simulink library "bcm"  (R2021b)
settings: Solver=VariableStepAuto  StartTime=0.0  StopTime=10.0  RelTol=1e-3
undefined symbols (not defined in the file or in its folder): ENUM_ANTITHEFT_ALARM, ENUM_ANTITHEFT_ARM, ENUM_ANTITHEFT_DISARM, ENUM_ANTITHEFT_WAIT, ENUM_GEARPOSNTOCAN_P, ENUM_PDKEYRAWLULOCK_INUNLOCK, ENUM_PDKEYRAWPS_INPS, ENUM_POWERSTA_ON, ENUM_POWERSTA_READY, ENUM_POWERSTA_STANDBY, ENUM_PWRSTASW_ON, ENUM_PWRSTASW_READY, ENUM_VEHICLETYPE_D21, ENUM_VEHICLETYPE_D31F25, ENUM_VEHICLETYPE_D31HAWD, ENUM_VEHICLETYPE_D31HRWD, ENUM_VEHICLETYPE_D31L24, FALSE, KBCM_ACCSwcPrsTmr_s, KBCM_ALMBrightnessDark_enum, KBCM_AmbBlue_enum, KBCM_AmbBreathT_ms, KBCM_AmbGreen_enum, KBCM_AmbMidPple_enum, KBCM_AmbRed_enum, KBCM_AmbTempCtrlEN_flg, KBCM_AmbTempT_s, KBCM_AmbWelModeENWait_s, KBCM_Antitheft_enum_ovrdflg, KBCM_Antitheft_enum_ovrdval, KBCM_APMDoorCtrlSta_flg_ovrdflg, KBCM_APMDoorCtrlSta_flg_ovrdval, KBCM_CmdKeepT_s, KBCM_CSWLightRstDebT_s, KBCM_CSWTurnLPRstT_s, KBCM_DelayTSW_flg, KBCM_DiagDRLOFF_flg, KBCM_DiagFLTC_mA, KBCM_DiagFMHT_s, KBCM_DiagFRTC_mA, KBCM_DiagRLTC_mA, KBCM_DiagRRTC_mA, KBCM_DrAPMRetryTimes_cnt, KBCM_DrOpenWdwOT_s, KBCM_DrOpenWdwReady_s, KBCM_ESSOffT_ms, KBCM_ESSOnT_ms, KBCM_FDCDKCReDetectT_K, KBCM_FDCDKCUSSFilterT_K, KBCM_HandleLampKeepT_s, KBCM_IVIRstHoldT_ms, KBCM_IVIRstTriggerT_ms, KBCM_ONDelayT_ms, KBCM_RAPSAbnFlashOFFT_ms, KBCM_RAPSAbnFlashONT_ms, KBCM_ReDetectT_K, KBCM_RightHandDriveEN_flg, KBCM_RLSLowSpdFilterT_s, KBCM_RmLampKeep_min, KBCM_RmLpKeyInT_s ... (+37)
libraries: simulink x389, $bdroot x11, hcu_lib x2
(part 7 of 13)

== system bcm/BCM/BCM/Window_Control_Sig_Combine/Driver_Window ==
  note: 0:NoReq
      | 1:BCM
      | 2.IVI
      | 3:DKC
      | 4:CONN
  note: 0:NoReq
      | 1:BCM
      | 2.IVI
      | 3:DKC
      | 4:CONN
  DKCWINCMD : Inport
  IVIWINCMD : Inport  Port=2
  CONNWINCMD : Inport  Port=3
  BCMWINCMD : Inport  Port=4
  Add{,1..3} (4 alike) : Sum  Inputs=-+
  Compare To Constant{,1..3} (4 alike) : simulink/Logic and Bit Operations/Compare To Constant  relop=>  const=0  OutDataTypeStr=boolean
  Constant{,1..3} (4 alike) : Constant  Value=100
  Constant10 : Constant  Value=127
  Constant{11,13,15,17} (4 alike) : Constant  Value=10
  Constant{8,12,14,16,18} (5 alike) : Constant
  Constant4 : Constant  Value=0
  Constant5 : Constant  Value=4
  Constant6 : Constant  Value=2
  Constant7 : Constant  Value=3
  Constant9 : Constant  Value=127
  Data Type Conversion{,1..6} (7 alike) : DataTypeConversion  OutDataTypeStr=uint8
  Data Type Conversion{7..14} (8 alike) : DataTypeConversion  OutDataTypeStr=int8
  Detect Decrease{1..4} (4 alike) : simulink/Logic and Bit Operations/Detect Decrease  vinit=0.0  OutDataTypeStr=boolean
  Multiport Switch : MultiPortSwitch  DataPortOrder=Zero-based contiguous  Inputs=6  DiagnosticForDefault=None  zeroidx=on
  Relational Operator{,1..3} (4 alike) : RelationalOperator  Operator=>  OutDataTypeStr=boolean  RndMeth=Simplest
  Saturation{,1..3} (4 alike) : Saturate  UpperLimit=10  LowerLimit=0
  Switch{,1..7} (8 alike) : Switch  Criteria=u2 > Threshold
  Unit Delay{,1..3} (4 alike) : UnitDelay  SampleTime=-1  HasFrameUpgradeWarning=on
  WINCMD : Outport
  WINReqAP : Outport  Port=2
  wires:
  Constant7/1 -> Data Type Conversion3/1
  CONNWINCMD/1 -> [CONNWINCMD]
  [CONNWINCMD] -> Relational Operator2/1
  Constant5/1 -> Data Type Conversion1/1
  [WINReqAP] -> Multiport Switch/1
  [BCMReq] -> Switch3/2
  Constant10/1 -> Data Type Conversion6/1
  [DKCReq] -> Switch1/2
  Constant9/1 -> Data Type Conversion5/1
  [CONNReq] -> Switch/2
  [DKCWINCMD] -> Multiport Switch/5
  Constant8/1 -> Data Type Conversion4/1
  Data Type Conversion/1 -> Switch/3
  [BCMWINCMD] -> Multiport Switch/3
  Multiport Switch/1 -> WINCMD/1
  Data Type Conversion3/1 -> Switch1/1
  Data Type Conversion1/1 -> Switch/1
  Constant2/1 -> Relational Operator2/2
  Constant4/1 -> Data Type Conversion/1
  Constant3/1 -> Relational Operator3/2
  Data Type Conversion5/1 -> Multiport Switch/2
  DKCWINCMD/1 -> [DKCWINCMD]
  BCMWINCMD/1 -> [BCMWINCMD]
  IVIWINCMD/1 -> [IVIWINCMD]
  Constant/1 -> Relational Operator/2
  [DKCWINCMD] -> Relational Operator/1
  [IVIWINCMD] -> Multiport Switch/4
  [CONNWINCMD] -> Multiport Switch/6
  Constant1/1 -> Relational Operator1/2
  [BCMWINCMD] -> Relational Operator3/1
  Data Type Conversion4/1 -> Switch3/1
  Switch1/1 -> Switch2/3
  Switch/1 -> Switch1/3
  [IVIWINCMD] -> Relational Operator1/1
  Switch3/1 -> [WINReqAP]
  Switch2/1 -> Switch3/3
  Constant6/1 -> Data Type Conversion2/1
  Data Type Conversion2/1 -> Switch2/1
  [IVIReq] -> Switch2/2
  [WINReqAP] -> WINReqAP/1
  Data Type Conversion6/1 -> Multiport Switch/7
  Relational Operator/1 -> Detect Decrease4/1
  Saturation/1 -> Compare To Constant/1, Unit Delay/1
  Constant11/1 -> Data Type Conversion7/1
  Detect Decrease4/1 -> Switch4/2
  Unit Delay/1 -> Add/2
  Add/1 -> Switch4/3
  Data Type Conversion7/1 -> Switch4/1
  Data Type Conversion8/1 -> Add/1
  Constant12/1 -> Data Type Conversion8/1
  Switch4/1 -> Saturation/1
  Compare To Constant/1 -> [DKCReq]
  Compare To Constant1/1 -> [IVIReq]
  Switch5/1 -> Saturation1/1
  Constant14/1 -> Data Type Conversion10/1
  Data Type Conversion10/1 -> Add1/1
  Data Type Conversion9/1 -> Switch5/1
  Add1/1 -> Switch5/3
  Unit Delay1/1 -> Add1/2
  Detect Decrease1/1 -> Switch5/2
  Constant13/1 -> Data Type Conversion9/1
  Saturation1/1 -> Unit Delay1/1, Compare To Constant1/1
  Relational Operator1/1 -> Detect Decrease1/1
  Saturation2/1 -> Compare To Constant2/1, Unit Delay2/1
  Constant15/1 -> Data Type Conversion12/1
  Detect Decrease2/1 -> Switch6/2
  Unit Delay2/1 -> Add2/2
  Add2/1 -> Switch6/3
  Data Type Conversion12/1 -> Switch6/1
  Data Type Conversion11/1 -> Add2/1
  Constant16/1 -> Data Type Conversion11/1
  Switch6/1 -> Saturation2/1
  Compare To Constant2/1 -> [CONNReq]
  Relational Operator2/1 -> Detect Decrease2/1
  Compare To Constant3/1 -> [BCMReq]
  Switch7/1 -> Saturation3/1
  Constant18/1 -> Data Type Conversion13/1
  Data Type Conversion13/1 -> Add3/1
  Data Type Conversion14/1 -> Switch7/1
  Add3/1 -> Switch7/3
  Unit Delay3/1 -> Add3/2
  Detect Decrease3/1 -> Switch7/2
  Constant17/1 -> Data Type Conversion14/1
  Saturation3/1 -> Unit Delay3/1, Compare To Constant3/1
  Relational Operator3/1 -> Detect Decrease3/1

== system bcm/BCM/BCM/Window_Control_Sig_Combine/Passenger_Window ==
  note: 0:NoReq
      | 1:BCM
      | 2.IVI
      | 3:DKC
      | 4:CONN
  note: 0:NoReq
      | 1:BCM
      | 2.IVI
      | 3:DKC
      | 4:CONN
  DKCWINCMD : Inport
  IVIWINCMD : Inport  Port=2
  CONNWINCMD : Inport  Port=3
  BCMWINCMD : Inport  Port=4
  Add{,1..3} (4 alike) : Sum  Inputs=-+
  Compare To Constant{,1..3} (4 alike) : simulink/Logic and Bit Operations/Compare To Constant  relop=>  const=0  OutDataTypeStr=boolean
  Constant{,1..3} (4 alike) : Constant  Value=100
  Constant10 : Constant  Value=127
  Constant{11,13,15,17} (4 alike) : Constant  Value=10
  Constant{8,12,14,16,18} (5 alike) : Constant
  Constant4 : Constant  Value=0
  Constant5 : Constant  Value=4
  Constant6 : Constant  Value=2
  Constant7 : Constant  Value=3
  Constant9 : Constant  Value=127
  Data Type Conversion{,1..6} (7 alike) : DataTypeConversion  OutDataTypeStr=uint8
  Data Type Conversion{7..14} (8 alike) : DataTypeConversion  OutDataTypeStr=int8
  Detect Decrease{1..4} (4 alike) : simulink/Logic and Bit Operations/Detect Decrease  vinit=0.0  OutDataTypeStr=boolean
  Multiport Switch : MultiPortSwitch  DataPortOrder=Zero-based contiguous  Inputs=6  DiagnosticForDefault=None  zeroidx=on
  Relational Operator{,1..3} (4 alike) : RelationalOperator  Operator=>  OutDataTypeStr=boolean  RndMeth=Simplest
  Saturation{,1..3} (4 alike) : Saturate  UpperLimit=10  LowerLimit=0
  Switch{,1..7} (8 alike) : Switch  Criteria=u2 > Threshold
  Unit Delay{,1..3} (4 alike) : UnitDelay  SampleTime=-1  HasFrameUpgradeWarning=on
  WINCMD : Outport
  WINReqAP : Outport  Port=2
  wires:
  Relational Operator3/1 -> Detect Decrease3/1
  Saturation3/1 -> Compare To Constant3/1, Unit Delay3/1
  Constant17/1 -> Data Type Conversion14/1
  Detect Decrease3/1 -> Switch7/2
  Unit Delay3/1 -> Add3/2
  Add3/1 -> Switch7/3
  Data Type Conversion14/1 -> Switch7/1
  Data Type Conversion13/1 -> Add3/1
  Constant18/1 -> Data Type Conversion13/1
  Switch7/1 -> Saturation3/1
  Compare To Constant3/1 -> [BCMReq]
  Relational Operator2/1 -> Detect Decrease2/1
  Compare To Constant2/1 -> [CONNReq]
  Switch6/1 -> Saturation2/1
  Constant16/1 -> Data Type Conversion11/1
  Data Type Conversion11/1 -> Add2/1
  Data Type Conversion12/1 -> Switch6/1
  Add2/1 -> Switch6/3
  Unit Delay2/1 -> Add2/2
  Detect Decrease2/1 -> Switch6/2
  Constant15/1 -> Data Type Conversion12/1
  Saturation2/1 -> Unit Delay2/1, Compare To Constant2/1
  Relational Operator1/1 -> Detect Decrease1/1
  Saturation1/1 -> Compare To Constant1/1, Unit Delay1/1
  Constant13/1 -> Data Type Conversion9/1
  Detect Decrease1/1 -> Switch5/2
  Unit Delay1/1 -> Add1/2
  Add1/1 -> Switch5/3
  Data Type Conversion9/1 -> Switch5/1
  Data Type Conversion10/1 -> Add1/1
  Constant14/1 -> Data Type Conversion10/1
  Switch5/1 -> Saturation1/1
  Compare To Constant1/1 -> [IVIReq]
  Compare To Constant/1 -> [DKCReq]
  Switch4/1 -> Saturation/1
  Constant12/1 -> Data Type Conversion8/1
  Data Type Conversion8/1 -> Add/1
  Data Type Conversion7/1 -> Switch4/1
  Add/1 -> Switch4/3
  Unit Delay/1 -> Add/2
  Detect Decrease4/1 -> Switch4/2
  Constant11/1 -> Data Type Conversion7/1
  Saturation/1 -> Unit Delay/1, Compare To Constant/1
  Relational Operator/1 -> Detect Decrease4/1
  Data Type Conversion6/1 -> Multiport Switch/7
  [WINReqAP] -> WINReqAP/1
  [IVIReq] -> Switch2/2
  Data Type Conversion2/1 -> Switch2/1
  Constant6/1 -> Data Type Conversion2/1
  Switch2/1 -> Switch3/3
  Switch3/1 -> [WINReqAP]
  [IVIWINCMD] -> Relational Operator1/1
  Switch/1 -> Switch1/3
  Switch1/1 -> Switch2/3
  Data Type Conversion4/1 -> Switch3/1
  [BCMWINCMD] -> Relational Operator3/1
  Constant1/1 -> Relational Operator1/2
  [CONNWINCMD] -> Multiport Switch/6
  [IVIWINCMD] -> Multiport Switch/4
  [DKCWINCMD] -> Relational Operator/1
  Constant/1 -> Relational Operator/2
  IVIWINCMD/1 -> [IVIWINCMD]
  BCMWINCMD/1 -> [BCMWINCMD]
  DKCWINCMD/1 -> [DKCWINCMD]
  Data Type Conversion5/1 -> Multiport Switch/2
  Constant3/1 -> Relational Operator3/2
  Constant4/1 -> Data Type Conversion/1
  Constant2/1 -> Relational Operator2/2
  Data Type Conversion1/1 -> Switch/1
  Data Type Conversion3/1 -> Switch1/1
  Multiport Switch/1 -> WINCMD/1
  [BCMWINCMD] -> Multiport Switch/3
  Data Type Conversion/1 -> Switch/3
  Constant8/1 -> Data Type Conversion4/1
  [DKCWINCMD] -> Multiport Switch/5
  [CONNReq] -> Switch/2
  Constant9/1 -> Data Type Conversion5/1
  [DKCReq] -> Switch1/2
  Constant10/1 -> Data Type Conversion6/1
  [BCMReq] -> Switch3/2
  [WINReqAP] -> Multiport Switch/1
  Constant5/1 -> Data Type Conversion1/1
  [CONNWINCMD] -> Relational Operator2/1
  CONNWINCMD/1 -> [CONNWINCMD]
  Constant7/1 -> Data Type Conversion3/1

== system bcm/BCM/BCM/Window_Control_Sig_Combine/RearLeft_Window ==
  note: 0:NoReq
      | 1:BCM
      | 2.IVI
      | 3:DKC
      | 4:CONN
  note: 0:NoReq
      | 1:BCM
      | 2.IVI
      | 3:DKC
      | 4:CONN
  DKCWINCMD : Inport
  IVIWINCMD : Inport  Port=2
  CONNWINCMD : Inport  Port=3
  BCMWINCMD : Inport  Port=4
  Add{,1..3} (4 alike) : Sum  Inputs=-+
  Compare To Constant{,1..3} (4 alike) : simulink/Logic and Bit Operations/Compare To Constant  relop=>  const=0  OutDataTypeStr=boolean
  Constant{,1..3} (4 alike) : Constant  Value=100
  Constant10 : Constant  Value=127
  Constant{11,13,15,17} (4 alike) : Constant  Value=10
  Constant{8,12,14,16,18} (5 alike) : Constant
  Constant4 : Constant  Value=0
  Constant5 : Constant  Value=4
  Constant6 : Constant  Value=2
  Constant7 : Constant  Value=3
  Constant9 : Constant  Value=127
  Data Type Conversion{,1..6} (7 alike) : DataTypeConversion  OutDataTypeStr=uint8
  Data Type Conversion{7..14} (8 alike) : DataTypeConversion  OutDataTypeStr=int8
  Detect Decrease{1..4} (4 alike) : simulink/Logic and Bit Operations/Detect Decrease  vinit=0.0  OutDataTypeStr=boolean
  Multiport Switch : MultiPortSwitch  DataPortOrder=Zero-based contiguous  Inputs=6  DiagnosticForDefault=None  zeroidx=on
  Relational Operator{,1..3} (4 alike) : RelationalOperator  Operator=>  OutDataTypeStr=boolean  RndMeth=Simplest
  Saturation{,1..3} (4 alike) : Saturate  UpperLimit=10  LowerLimit=0
  Switch{,1..7} (8 alike) : Switch  Criteria=u2 > Threshold
  Unit Delay{,1..3} (4 alike) : UnitDelay  SampleTime=-1  HasFrameUpgradeWarning=on
  WINCMD : Outport
  WINReqAP : Outport  Port=2
  wires:
  Relational Operator3/1 -> Detect Decrease3/1
  Saturation3/1 -> Compare To Constant3/1, Unit Delay3/1
  Constant17/1 -> Data Type Conversion14/1
  Detect Decrease3/1 -> Switch7/2
  Unit Delay3/1 -> Add3/2
  Add3/1 -> Switch7/3
  Data Type Conversion14/1 -> Switch7/1
  Data Type Conversion13/1 -> Add3/1
  Constant18/1 -> Data Type Conversion13/1
  Switch7/1 -> Saturation3/1
  Compare To Constant3/1 -> [BCMReq]
  Relational Operator2/1 -> Detect Decrease2/1
  Compare To Constant2/1 -> [CONNReq]
  Switch6/1 -> Saturation2/1
  Constant16/1 -> Data Type Conversion11/1
  Data Type Conversion11/1 -> Add2/1
  Data Type Conversion12/1 -> Switch6/1
  Add2/1 -> Switch6/3
  Unit Delay2/1 -> Add2/2
  Detect Decrease2/1 -> Switch6/2
  Constant15/1 -> Data Type Conversion12/1
  Saturation2/1 -> Unit Delay2/1, Compare To Constant2/1
  Relational Operator1/1 -> Detect Decrease1/1
  Saturation1/1 -> Compare To Constant1/1, Unit Delay1/1
  Constant13/1 -> Data Type Conversion9/1
  Detect Decrease1/1 -> Switch5/2
  Unit Delay1/1 -> Add1/2
  Add1/1 -> Switch5/3
  Data Type Conversion9/1 -> Switch5/1
  Data Type Conversion10/1 -> Add1/1
  Constant14/1 -> Data Type Conversion10/1
  Switch5/1 -> Saturation1/1
  Compare To Constant1/1 -> [IVIReq]
  Compare To Constant/1 -> [DKCReq]
  Switch4/1 -> Saturation/1
  Constant12/1 -> Data Type Conversion8/1
  Data Type Conversion8/1 -> Add/1
  Data Type Conversion7/1 -> Switch4/1
  Add/1 -> Switch4/3
  Unit Delay/1 -> Add/2
  Detect Decrease4/1 -> Switch4/2
  Constant11/1 -> Data Type Conversion7/1
  Saturation/1 -> Unit Delay/1, Compare To Constant/1
  Relational Operator/1 -> Detect Decrease4/1
  Data Type Conversion6/1 -> Multiport Switch/7
  [WINReqAP] -> WINReqAP/1
  [IVIReq] -> Switch2/2
  Data Type Conversion2/1 -> Switch2/1
  Constant6/1 -> Data Type Conversion2/1
  Switch2/1 -> Switch3/3
  Switch3/1 -> [WINReqAP]
  [IVIWINCMD] -> Relational Operator1/1
  Switch/1 -> Switch1/3
  Switch1/1 -> Switch2/3
  Data Type Conversion4/1 -> Switch3/1
  [BCMWINCMD] -> Relational Operator3/1
  Constant1/1 -> Relational Operator1/2
  [CONNWINCMD] -> Multiport Switch/6
  [IVIWINCMD] -> Multiport Switch/4
  [DKCWINCMD] -> Relational Operator/1
  Constant/1 -> Relational Operator/2
  IVIWINCMD/1 -> [IVIWINCMD]
  BCMWINCMD/1 -> [BCMWINCMD]
  DKCWINCMD/1 -> [DKCWINCMD]
  Data Type Conversion5/1 -> Multiport Switch/2
  Constant3/1 -> Relational Operator3/2
  Constant4/1 -> Data Type Conversion/1
  Constant2/1 -> Relational Operator2/2
  Data Type Conversion1/1 -> Switch/1
  Data Type Conversion3/1 -> Switch1/1
  Multiport Switch/1 -> WINCMD/1
  [BCMWINCMD] -> Multiport Switch/3
  Data Type Conversion/1 -> Switch/3
  Constant8/1 -> Data Type Conversion4/1
  [DKCWINCMD] -> Multiport Switch/5
  [CONNReq] -> Switch/2
  Constant9/1 -> Data Type Conversion5/1
  [DKCReq] -> Switch1/2
  Constant10/1 -> Data Type Conversion6/1
  [BCMReq] -> Switch3/2
  [WINReqAP] -> Multiport Switch/1
  Constant5/1 -> Data Type Conversion1/1
  [CONNWINCMD] -> Relational Operator2/1
  CONNWINCMD/1 -> [CONNWINCMD]
  Constant7/1 -> Data Type Conversion3/1

== system bcm/BCM/BCM/Window_Control_Sig_Combine/RearRight_Window ==
  note: 0:NoReq
      | 1:BCM
      | 2.IVI
      | 3:DKC
      | 4:CONN
  note: 0:NoReq
      | 1:BCM
      | 2.IVI
      | 3:DKC
      | 4:CONN
  DKCWINCMD : Inport
  IVIWINCMD : Inport  Port=2
  CONNWINCMD : Inport  Port=3
  BCMWINCMD : Inport  Port=4
  Add{,1..3} (4 alike) : Sum  Inputs=-+
  Compare To Constant{,1..3} (4 alike) : simulink/Logic and Bit Operations/Compare To Constant  relop=>  const=0  OutDataTypeStr=boolean
  Constant{,1..3} (4 alike) : Constant  Value=100
  Constant10 : Constant  Value=127
  Constant{11,13,15,17} (4 alike) : Constant  Value=10
  Constant{8,12,14,16,18} (5 alike) : Constant
  Constant4 : Constant  Value=0
  Constant5 : Constant  Value=4
  Constant6 : Constant  Value=2
  Constant7 : Constant  Value=3
  Constant9 : Constant  Value=127
  Data Type Conversion{,1..6} (7 alike) : DataTypeConversion  OutDataTypeStr=uint8
  Data Type Conversion{7..14} (8 alike) : DataTypeConversion  OutDataTypeStr=int8
  Detect Decrease{1..4} (4 alike) : simulink/Logic and Bit Operations/Detect Decrease  vinit=0.0  OutDataTypeStr=boolean
  Multiport Switch : MultiPortSwitch  DataPortOrder=Zero-based contiguous  Inputs=6  DiagnosticForDefault=None  zeroidx=on
  Relational Operator{,1..3} (4 alike) : RelationalOperator  Operator=>  OutDataTypeStr=boolean  RndMeth=Simplest
  Saturation{,1..3} (4 alike) : Saturate  UpperLimit=10  LowerLimit=0
  Switch{,1..7} (8 alike) : Switch  Criteria=u2 > Threshold
  Unit Delay{,1..3} (4 alike) : UnitDelay  SampleTime=-1  HasFrameUpgradeWarning=on
  WINCMD : Outport
  WINReqAP : Outport  Port=2
  wires:
  Constant7/1 -> Data Type Conversion3/1
  CONNWINCMD/1 -> [CONNWINCMD]
  [CONNWINCMD] -> Relational Operator2/1
  Constant5/1 -> Data Type Conversion1/1
  [WINReqAP] -> Multiport Switch/1
  [BCMReq] -> Switch3/2
  Constant10/1 -> Data Type Conversion6/1
  [DKCReq] -> Switch1/2
  Constant9/1 -> Data Type Conversion5/1
  [CONNReq] -> Switch/2
  [DKCWINCMD] -> Multiport Switch/5
  Constant8/1 -> Data Type Conversion4/1
  Data Type Conversion/1 -> Switch/3
  [BCMWINCMD] -> Multiport Switch/3
  Multiport Switch/1 -> WINCMD/1
  Data Type Conversion3/1 -> Switch1/1
  Data Type Conversion1/1 -> Switch/1
  Constant2/1 -> Relational Operator2/2
  Constant4/1 -> Data Type Conversion/1
  Constant3/1 -> Relational Operator3/2
  Data Type Conversion5/1 -> Multiport Switch/2
  DKCWINCMD/1 -> [DKCWINCMD]
  BCMWINCMD/1 -> [BCMWINCMD]
  IVIWINCMD/1 -> [IVIWINCMD]
  Constant/1 -> Relational Operator/2
  [DKCWINCMD] -> Relational Operator/1
  [IVIWINCMD] -> Multiport Switch/4
  [CONNWINCMD] -> Multiport Switch/6
  Constant1/1 -> Relational Operator1/2
  [BCMWINCMD] -> Relational Operator3/1
  Data Type Conversion4/1 -> Switch3/1
  Switch1/1 -> Switch2/3
  Switch/1 -> Switch1/3
  [IVIWINCMD] -> Relational Operator1/1
  Switch3/1 -> [WINReqAP]
  Switch2/1 -> Switch3/3
  Constant6/1 -> Data Type Conversion2/1
  Data Type Conversion2/1 -> Switch2/1
  [IVIReq] -> Switch2/2
  [WINReqAP] -> WINReqAP/1
  Data Type Conversion6/1 -> Multiport Switch/7
  Relational Operator/1 -> Detect Decrease4/1
  Saturation/1 -> Compare To Constant/1, Unit Delay/1
  Constant11/1 -> Data Type Conversion7/1
  Detect Decrease4/1 -> Switch4/2
  Unit Delay/1 -> Add/2
  Add/1 -> Switch4/3
  Data Type Conversion7/1 -> Switch4/1
  Data Type Conversion8/1 -> Add/1
  Constant12/1 -> Data Type Conversion8/1
  Switch4/1 -> Saturation/1
  Compare To Constant/1 -> [DKCReq]
  Compare To Constant1/1 -> [IVIReq]
  Switch5/1 -> Saturation1/1
  Constant14/1 -> Data Type Conversion10/1
  Data Type Conversion10/1 -> Add1/1
  Data Type Conversion9/1 -> Switch5/1
  Add1/1 -> Switch5/3
  Unit Delay1/1 -> Add1/2
  Detect Decrease1/1 -> Switch5/2
  Constant13/1 -> Data Type Conversion9/1
  Saturation1/1 -> Unit Delay1/1, Compare To Constant1/1
  Relational Operator1/1 -> Detect Decrease1/1
  Saturation2/1 -> Compare To Constant2/1, Unit Delay2/1
  Constant15/1 -> Data Type Conversion12/1
  Detect Decrease2/1 -> Switch6/2
  Unit Delay2/1 -> Add2/2
  Add2/1 -> Switch6/3
  Data Type Conversion12/1 -> Switch6/1
  Data Type Conversion11/1 -> Add2/1
  Constant16/1 -> Data Type Conversion11/1
  Switch6/1 -> Saturation2/1
  Compare To Constant2/1 -> [CONNReq]
  Relational Operator2/1 -> Detect Decrease2/1
  Compare To Constant3/1 -> [BCMReq]
  Switch7/1 -> Saturation3/1
  Constant18/1 -> Data Type Conversion13/1
  Data Type Conversion13/1 -> Add3/1
  Data Type Conversion14/1 -> Switch7/1
  Add3/1 -> Switch7/3
  Unit Delay3/1 -> Add3/2
  Detect Decrease3/1 -> Switch7/2
  Constant17/1 -> Data Type Conversion14/1
  Saturation3/1 -> Unit Delay3/1, Compare To Constant3/1
  Relational Operator3/1 -> Detect Decrease3/1

== system bcm/BCM/BCM/PTG/KeyDetected/CheckSignalAvailable ==
  VBCM_PASDRML_cm_IN : Inport
  VBCM_PASDRMR_cm_IN : Inport  Port=2
  KBCM_USSDis_cm_IN : Inport  Port=3
  AND : Logic  Inputs=3  AllPortsSameDT=off  OutDataTypeStr=boolean
  Constant : Constant  OutDataTypeStr=single
  Constant1 : Constant  OutDataTypeStr=single
  Constant2 : Constant  OutDataTypeStr=single
  Constant3 : Constant  Value=KBCM_SPTGLowerBound_cm
  Constant4 : Constant  Value=KBCM_SPTGLowerBoundOut_cm
  Constant5 : Constant  Value=KBCM_SPTGLowerBound_cm
  Constant6 : Constant  Value=KBCM_SPTGLowerBoundOut_cm
  Demux : Demux  Outputs=3
  Equal : RelationalOperator  OutDataTypeStr=boolean  RndMeth=Simplest
  Equal1 : RelationalOperator  OutDataTypeStr=boolean  RndMeth=Simplest
  GreaterThan : RelationalOperator  OutDataTypeStr=boolean  RndMeth=Simplest
  Max : MinMax  Function=max  Inputs=3
  Mux : Mux  Inputs=3
  Mux1 : Mux  Inputs=3
  Sum : Sum  Inputs=+-
  Sum1 : Sum  Inputs=+++
  Sum2 : Sum  Inputs=|+-
  Sum3 : Sum  Inputs=|+-
  Switch : Switch  Criteria=u2 > Threshold
  VBCM_PASDRML_cm : Outport
  VBCM_PASDRMR_cm : Outport  Port=2
  KBCM_USSDis_cm : Outport  Port=3
  CheckResult : Outport  Port=4
  wires:
  GreaterThan/1 -> AND/1
  VBCM_PASDRML_cm_IN/1 -> [VBCM_PASDRML_cm_IN]
  VBCM_PASDRMR_cm_IN/1 -> [VBCM_PASDRMR_cm_IN]
  KBCM_USSDis_cm_IN/1 -> [KBCM_USSDis_cm_IN]
  AND/1 -> Switch/2, CheckResult/1
  Mux/1 -> Switch/1
  [VBCM_PASDRML_cm_IN] -> Mux/1
  [VBCM_PASDRMR_cm_IN] -> Mux/2
  [KBCM_USSDis_cm_IN] -> Mux/3
  Mux1/1 -> Switch/3
  Constant/1 -> Mux1/1
  Constant1/1 -> Mux1/2
  Switch/1 -> Demux/1
  Demux/1 -> VBCM_PASDRML_cm/1
  Demux/2 -> VBCM_PASDRMR_cm/1
  Demux/3 -> KBCM_USSDis_cm/1
  Equal/1 -> AND/2
  [VBCM_PASDRML_cm_IN] -> Max/1, Sum1/1
  [VBCM_PASDRMR_cm_IN] -> Max/2, Sum1/2
  [KBCM_USSDis_cm_IN] -> Max/3, Sum1/3
  Sum1/1 -> Sum/1
  Max/1 -> Sum/2, GreaterThan/2
  Sum/1 -> GreaterThan/1
  Constant2/1 -> Mux1/3
  Equal1/1 -> AND/3
  [VBCM_PASDRMR_cm_IN] -> Equal/1
  Constant3/1 -> Sum2/1
  Constant4/1 -> Sum2/2
  Sum2/1 -> Equal/2
  Sum3/1 -> Equal1/2
  Constant6/1 -> Sum3/2
  Constant5/1 -> Sum3/1
  [VBCM_PASDRML_cm_IN] -> Equal1/1

== system bcm/BCM/BCM/PTG/KeyDetected/Target_h ==
  VBCM_PASDRML_cm : Inport
  VBCM_PASDRMR_cm : Inport  Port=2
  KBCM_USSDis_cm : Inport  Port=3
  Data Type Conversion : DataTypeConversion
  Divide : Product  Inputs=*/
  Gain : Gain  Gain=2
  Gain1 : Gain  Gain=0.5
  Product : Product  Inputs=4
  Sqrt1 : Sqrt  SaturateOnIntegerOverflow=on
  Sum : Sum  Inputs=+-
  Sum1 : Sum  Inputs=+++
  Sum2 : Sum  Inputs=+-
  Sum3 : Sum  Inputs=+-
  Terminator : Terminator
  Target_h : Outport
  wires:
  Divide/1 -> Data Type Conversion/1, Target_h/1
  VBCM_PASDRML_cm/1 -> Sum/2, Sum1/1
  VBCM_PASDRMR_cm/1 -> Sum2/2, Sum1/2
  KBCM_USSDis_cm/1 -> Divide/2, Sum3/2, Sum1/3
  Sum1/1 -> Gain1/1
  Sum/1 -> Product/2
  Sum2/1 -> Product/3
  Sum3/1 -> Product/4
  Product/1 -> Sqrt1/1
  Sqrt1/1 -> Gain/1
  Gain/1 -> Divide/1
  Gain1/1 -> Sum3/1, Sum2/1, Sum/1, Product/1
  Data Type Conversion/1 -> Terminator/1  "VBCM_Targeth_cm"

== system bcm/BCM/BCM/PTG/KeyDetected/cosRML ==
  VBCM_PASDRML_cm : Inport
  VBCM_PASDRMR_cm : Inport  Port=2
  KBCM_USSDis_cm : Inport  Port=3
  Divide : Product  Inputs=*/
  Gain : Gain  Gain=2
  Product : Product
  Square : Math  Operator=square  SaturateOnIntegerOverflow=on
  Square1 : Math  Operator=square  SaturateOnIntegerOverflow=on
  Square2 : Math  Operator=square  SaturateOnIntegerOverflow=on
  Sum : Sum  Inputs=+-+
  cosRML : Outport
  wires:
  VBCM_PASDRML_cm/1 -> Product/1, Square/1
  VBCM_PASDRMR_cm/1 -> Square1/1
  KBCM_USSDis_cm/1 -> Product/2, Square2/1
  Square/1 -> Sum/1
  Square1/1 -> Sum/2
  Square2/1 -> Sum/3
  Product/1 -> Gain/1
  Sum/1 -> Divide/1
  Divide/1 -> cosRML/1
  Gain/1 -> Divide/2

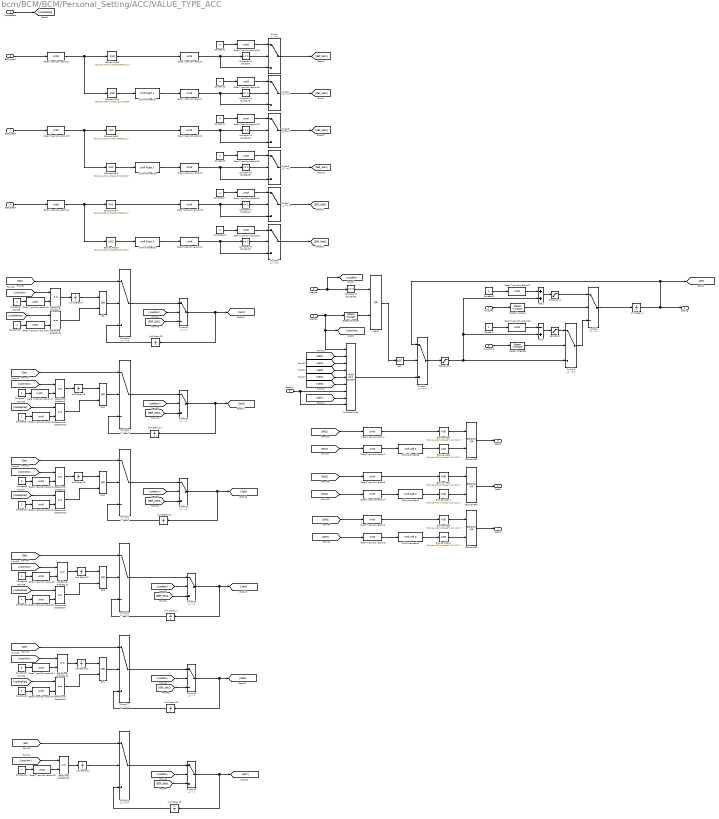
== system bcm/BCM/BCM/Personal_Setting/ACC/VALUE_TYPE_ACC ==
  UserNow : Inport
  Loadbar : Inport  Port=2
  UpdateReq : Inport  Port=3
  PlusCmd : Inport  Port=4
  MinusCmd : Inport  Port=5
  EEP_Set12 : Inport  Port=6
  EEP_Set34 : Inport  Port=7
  EEP_Set57 : Inport  Port=8
  Default : Inport  Port=9
  AND11 : Logic  Operator=OR  AllPortsSameDT=off  OutDataTypeStr=boolean
  Add : Sum  Inputs=-+
  Add1 : Sum
  Bitwise AND{1..4,11..12} (6 alike) : simulink/Logic and Bit Operations/Bitwise Operator  logicop=AND  UseBitMask=on  BitMask=bin2dec('11111111')  BitMaskRealWorld=Stored Integer
  Bitwise AND10 : simulink/Logic and Bit Operations/Bitwise Operator  logicop=AND  UseBitMask=on  BitMask=bin2dec('00111000')  BitMaskRealWorld=Stored Integer
  Bitwise AND5 : simulink/Logic and Bit Operations/Bitwise Operator  logicop=AND  UseBitMask=on  BitMask=bin2dec('00000111')  BitMaskRealWorld=Stored Integer
  Bitwise AND6 : simulink/Logic and Bit Operations/Bitwise Operator  logicop=AND  UseBitMask=on  BitMask=bin2dec('00111000')  BitMaskRealWorld=Stored Integer
  Bitwise AND7 : simulink/Logic and Bit Operations/Bitwise Operator  logicop=AND  UseBitMask=on  BitMask=bin2dec('00000111')  BitMaskRealWorld=Stored Integer
  Bitwise AND8 : simulink/Logic and Bit Operations/Bitwise Operator  logicop=AND  UseBitMask=on  BitMask=bin2dec('00000111')  BitMaskRealWorld=Stored Integer
  Bitwise AND9 : simulink/Logic and Bit Operations/Bitwise Operator  logicop=AND  UseBitMask=on  BitMask=bin2dec('00111000')  BitMaskRealWorld=Stored Integer
  Bitwise OR1 : simulink/Logic and Bit Operations/Bitwise Operator  logicop=OR  UseBitMask=off  NumInputPorts=2  BitMask=bin2dec('00000000000000000000')  BitMaskRealWorld=Stored Integer
  Bitwise OR2 : simulink/Logic and Bit Operations/Bitwise Operator  logicop=OR  UseBitMask=off  NumInputPorts=2  BitMask=bin2dec('00000000000000000000')  BitMaskRealWorld=Stored Integer
  Bitwise OR3 : simulink/Logic and Bit Operations/Bitwise Operator  logicop=OR  UseBitMask=off  NumInputPorts=2  BitMask=bin2dec('00000000000000000000')  BitMaskRealWorld=Stored Integer
  Compare To Constant{,1..4,6} (6 alike) : simulink/Logic and Bit Operations/Compare To Constant  relop=<=  const=0  OutDataTypeStr=boolean
  Compare To Constant5 : simulink/Logic and Bit Operations/Compare To Constant  relop===  const=0  OutDataTypeStr=boolean
  Constant : Constant
  Constant1 : Constant
  Constant10 : Constant  Value=5  OutDataTypeStr=uint8
  Constant11 : Constant  Value=5  OutDataTypeStr=uint8
  Constant12 : Constant  Value=7  OutDataTypeStr=uint8
  Constant13 : Constant  OutDataTypeStr=uint8
  Constant14 : Constant  Value=2  OutDataTypeStr=uint8
  Constant15 : Constant  Value=3  OutDataTypeStr=uint8
  Constant16 : Constant  Value=4  OutDataTypeStr=uint8
  Constant{2..5,17..18} (6 alike) : Constant  Value=4
  Constant6 : Constant  OutDataTypeStr=uint8
  Constant7 : Constant  Value=2  OutDataTypeStr=uint8
  Constant8 : Constant  Value=3  OutDataTypeStr=uint8
  Constant9 : Constant  Value=4  OutDataTypeStr=uint8
  Data Type Conversion{,1..33} (34 alike) : DataTypeConversion  OutDataTypeStr=uint8
  Detect Change7 : simulink/Logic and Bit Operations/Detect Change  vinit=0  OutDataTypeStr=boolean
  Detect Increase : simulink/Logic and Bit Operations/Detect Increase  vinit=0.0  OutDataTypeStr=boolean
  Detect Increase1 : simulink/Logic and Bit Operations/Detect Increase  vinit=0.0  OutDataTypeStr=boolean
  Multiport Switch : MultiPortSwitch  Inputs=7  DataPortForDefault=Additional data port  DiagnosticForDefault=None
  NOT : Logic  Operator=NOT  IconShape=distinctive  AllPortsSameDT=off  OutDataTypeStr=boolean
  OR{,1..4} (5 alike) : Logic  Operator=OR  AllPortsSameDT=off  OutDataTypeStr=boolean
  Relational Operator{7..17} (11 alike) : RelationalOperator  Operator===  OutDataTypeStr=boolean  RndMeth=Simplest
  Saturation : Saturate  UpperLimit=4  LowerLimit=1
  Saturation1 : Saturate  UpperLimit=4  LowerLimit=1
  Saturation2 : Saturate  UpperLimit=4  LowerLimit=1
  Shift Arithmetic1 : ArithShift  BitShiftNumber=3  BitShiftDirection=Left
  Shift Arithmetic2 : ArithShift  BitShiftNumber=3  BitShiftDirection=Left
  Shift Arithmetic3 : ArithShift  BitShiftNumber=3  BitShiftDirection=Right
  Shift Arithmetic4 : ArithShift  BitShiftNumber=3  BitShiftDirection=Right
  Shift Arithmetic5 : ArithShift  BitShiftNumber=3  BitShiftDirection=Right
  Shift Arithmetic6 : ArithShift  BitShiftNumber=3  BitShiftDirection=Left
  Switch{,1..8,16..19,21,23} (15 alike) : Switch  Criteria=u2 ~= 0
  Switch{14..15,20,22,24..25} (6 alike) : Switch  Criteria=u2 > Threshold
  Unit Delay{1,14..25} (13 alike) : UnitDelay  SampleTime=-1  HasFrameUpgradeWarning=on
  Setting : Outport
  Set12 : Outport  Port=2
  Set34 : Outport  Port=3
  Set57 : Outport  Port=4
  wires:
  Saturation1/1 -> Switch2/1
  Saturation/1 -> Switch3/1
  Add1/1 -> Saturation1/1
  Constant1/1 -> Data Type Conversion27/1
  Data Type Conversion27/1 -> Add1/1
  Data Type Conversion26/1 -> Add/1
  Add/1 -> Saturation/1
  Constant/1 -> Data Type Conversion26/1
  Switch3/1 -> Switch2/3
  Detect Increase1/1 -> Switch3/2
  Detect Increase/1 -> Switch2/2
  MinusCmd/1 -> Detect Increase1/1
  PlusCmd/1 -> Detect Increase/1
  Default/1 -> Multiport Switch/7, Multiport Switch/9
  [Set7] -> Multiport Switch/8
  [Set5] -> Multiport Switch/6
  [Set4] -> Multiport Switch/5
  [Set3] -> Multiport Switch/4
  [Set2] -> Multiport Switch/3
  [Set1] -> Multiport Switch/2
  NOT/1 -> Switch1/2
  Detect Change7/1 -> AND11/2
  Multiport Switch/1 -> Switch1/3
  Switch1/1 -> Saturation2/1
  AND11/1 -> NOT/1
  Compare To Constant5/1 -> AND11/1
  UserNow/1 -> Multiport Switch/1, [UserNow], Detect Change7/1
  Loadbar/1 -> [Loadbar], Compare To Constant5/1
  Switch2/1 -> Unit Delay1/1
  Unit Delay1/1 -> Setting/1, Switch1/1, [Set]
  Bitwise AND1/1 -> Bitwise OR1/1
  Shift Arithmetic6/1 -> Bitwise AND2/1
  Data Type Conversion/1 -> Bitwise AND4/1
  Data Type Conversion3/1 -> Bitwise AND1/1
  Shift Arithmetic1/1 -> Bitwise AND11/1
  Data Type Conversion4/1 -> Shift Arithmetic1/1
  Bitwise AND2/1 -> Bitwise OR2/2
  Data Type Conversion1/1 -> Shift Arithmetic6/1
  Bitwise AND11/1 -> Bitwise OR1/2
  Bitwise AND4/1 -> Bitwise OR2/1
  Bitwise OR2/1 -> Set12/1
  Bitwise OR1/1 -> Set34/1
  [Set1] -> Data Type Conversion/1
  [Set2] -> Data Type Conversion1/1
  EEP_Set34/1 -> Data Type Conversion13/1
  [Set3] -> Data Type Conversion3/1
  [Set4] -> Data Type Conversion4/1
  [Set7] -> Data Type Conversion5/1
  [Set5] -> Data Type Conversion2/1
  Bitwise OR3/1 -> Set57/1
  Bitwise AND12/1 -> Bitwise OR3/2
  Data Type Conversion5/1 -> Shift Arithmetic2/1
  Shift Arithmetic2/1 -> Bitwise AND12/1
  Data Type Conversion2/1 -> Bitwise AND3/1
  Bitwise AND3/1 -> Bitwise OR3/1
  EEP_Set57/1 -> Data Type Conversion14/1
  EEP_Set12/1 -> Data Type Conversion12/1
  UpdateReq/1 -> [UpdateReq]
  Relational Operator10/1 -> OR4/2
  Data Type Conversion23/1 -> Relational Operator11/2
  Unit Delay21/1 -> OR4/1
  Relational Operator15/1 -> OR1/2
  Switch14/1 -> Unit Delay18/1, [Set5]
  Switch16/1 -> Switch15/1
  Switch15/1 -> Unit Delay19/1, [Set7]
  Constant10/1 -> Data Type Conversion22/1
  Relational Operator13/1 -> Unit Delay22/1
  Relational Operator9/1 -> Unit Delay15/1
  Unit Delay22/1 -> Switch16/2
  Switch19/1 -> Switch20/1
  [UpdateReq] -> Relational Operator14/1
  Relational Operator12/1 -> Unit Delay21/1
  [Loadbar] -> Switch14/2
  [EEP_Set1] -> Switch24/3
  Switch21/1 -> Switch22/1
  Switch17/1 -> Switch14/1
  Unit Delay14/1 -> Switch19/3
  Switch20/1 -> Unit Delay14/1, [Set2]
  [EEP_Set6] -> Switch15/3
  Constant9/1 -> Data Type Conversion23/1
  [Set] -> Switch18/1
  [EEP_Set4] -> Switch25/3
  [UserNow] -> Relational Operator11/1
  Unit Delay18/1 -> Switch17/3
  Switch23/1 -> Switch25/1
  Constant12/1 -> Data Type Conversion25/1
  [Set] -> Switch17/1
  [Loadbar] -> Switch20/2
  Relational Operator11/1 -> Unit Delay20/1
  Switch25/1 -> Unit Delay17/1, [Set4]
  [UserNow] -> Relational Operator13/1
  OR3/1 -> Switch23/2
  [Set] -> Switch19/1
  Constant7/1 -> Data Type Conversion17/1
  Data Type Conversion25/1 -> Relational Operator13/2
  [Loadbar] -> Switch22/2
  Constant6/1 -> Data Type Conversion15/1
  [UserNow] -> Relational Operator7/1
  [Loadbar] -> Switch15/2
  [Set] -> Switch21/1
  [Set] -> Switch23/1
  [Loadbar] -> Switch25/2
  [UserNow] -> Relational Operator9/1
  Relational Operator8/1 -> Unit Delay25/1
  Data Type Conversion16/1 -> Relational Operator14/2
  Unit Delay25/1 -> OR1/1
  Switch24/1 -> Unit Delay23/1, [Set1]
  [Loadbar] -> Switch24/2
  [UserNow] -> Relational Operator12/1
  Data Type Conversion24/1 -> Relational Operator12/2
  [Set] -> Switch16/1
  Unit Delay16/1 -> Switch21/3
  [UpdateReq] -> Relational Operator15/1
  Constant8/1 -> Data Type Conversion20/1
  Data Type Conversion18/1 -> Relational Operator15/2
  OR1/1 -> Switch19/2
  Data Type Conversion17/1 -> Relational Operator8/2
  Constant14/1 -> Data Type Conversion18/1
  [UpdateReq] -> Relational Operator16/1
  Relational Operator16/1 -> OR2/2
  Data Type Conversion21/1 -> Relational Operator17/2
  Constant11/1 -> Data Type Conversion24/1
  Unit Delay15/1 -> OR2/1
  Data Type Conversion22/1 -> Relational Operator10/2
  Relational Operator17/1 -> OR3/2
  Unit Delay20/1 -> OR3/1
  Switch18/1 -> Switch24/1
  Switch22/1 -> Unit Delay16/1, [Set3]
  [UpdateReq] -> Relational Operator17/1
  [UpdateReq] -> Relational Operator10/1
  Constant15/1 -> Data Type Conversion19/1
  Constant16/1 -> Data Type Conversion21/1
  Unit Delay17/1 -> Switch23/3
  Data Type Conversion19/1 -> Relational Operator16/2
  [EEP_Set3] -> Switch22/3
  Data Type Conversion15/1 -> Relational Operator7/2
  [UserNow] -> Relational Operator8/1
  [EEP_Set2] -> Switch20/3
  OR/1 -> Switch18/2
  [EEP_Set5] -> Switch14/3
  Relational Operator14/1 -> OR/2
  Relational Operator7/1 -> Unit Delay24/1
  OR4/1 -> Switch17/2
  Unit Delay24/1 -> OR/1
  Data Type Conversion20/1 -> Relational Operator9/2
  OR2/1 -> Switch21/2
  Unit Delay23/1 -> Switch18/3
  Unit Delay19/1 -> Switch16/3
  Constant13/1 -> Data Type Conversion16/1
  Bitwise AND10/1 -> Shift Arithmetic5/1
  Constant3/1 -> Data Type Conversion29/1
  Bitwise AND5/1 -> Data Type Conversion8/1
  Compare To Constant2/1 -> Switch5/2
  Switch/1 -> [EEP_Set1]
  Data Type Conversion8/1 -> Switch5/3, Compare To Constant2/1
  Data Type Conversion28/1 -> Switch/1
  Data Type Conversion9/1 -> Compare To Constant3/1, Switch6/3
  Bitwise AND8/1 -> Data Type Conversion6/1
  Switch4/1 -> [EEP_Set2]
  Switch8/1 -> [EEP_Set6]
  Constant4/1 -> Data Type Conversion30/1
  Data Type Conversion29/1 -> Switch4/1
  Shift Arithmetic3/1 -> Data Type Conversion9/1
  Switch5/1 -> [EEP_Set3]
  Compare To Constant6/1 -> Switch8/2
  Data Type Conversion33/1 -> Switch8/1
  Data Type Conversion30/1 -> Switch5/1
  Data Type Conversion10/1 -> Switch7/3, Compare To Constant4/1
  Switch7/1 -> [EEP_Set5]
  Compare To Constant/1 -> Switch/2
  Compare To Constant3/1 -> Switch6/2
  Bitwise AND9/1 -> Shift Arithmetic4/1
  Data Type Conversion32/1 -> Switch7/1
  Shift Arithmetic4/1 -> Data Type Conversion7/1
  Constant5/1 -> Data Type Conversion31/1
  Shift Arithmetic5/1 -> Data Type Conversion11/1
  Bitwise AND6/1 -> Shift Arithmetic3/1
  Switch6/1 -> [EEP_Set4]
  Constant2/1 -> Data Type Conversion28/1
  Bitwise AND7/1 -> Data Type Conversion10/1
  Constant17/1 -> Data Type Conversion32/1
  Data Type Conversion12/1 -> Bitwise AND8/1, Bitwise AND9/1
  Data Type Conversion7/1 -> Compare To Constant1/1, Switch4/3
  Compare To Constant4/1 -> Switch7/2
  Data Type Conversion13/1 -> Bitwise AND5/1, Bitwise AND6/1
  Data Type Conversion6/1 -> Switch/3, Compare To Constant/1
  Data Type Conversion14/1 -> Bitwise AND7/1, Bitwise AND10/1
  Constant18/1 -> Data Type Conversion33/1
  Data Type Conversion11/1 -> Compare To Constant6/1, Switch8/3
  Compare To Constant1/1 -> Switch4/2
  Data Type Conversion31/1 -> Switch6/1
  Saturation2/1 -> Switch3/3, Add1/2, Add/2

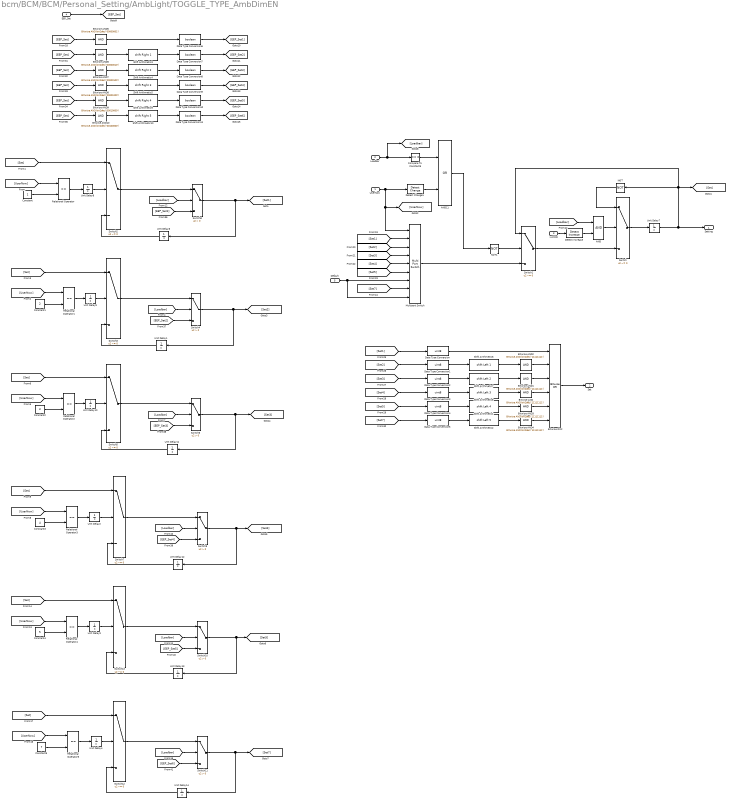
== system bcm/BCM/BCM/Personal_Setting/AmbLight/TOGGLE_TYPE_AmbDimEN ==
  UserNow : Inport
  Loadbar : Inport  Port=2
  iviCMD : Inport  Port=3
  EEP_Set : Inport  Port=4
  Default : Inport  Port=5
  AND : Logic  AllPortsSameDT=off  OutDataTypeStr=boolean
  AND11 : Logic  Operator=OR  AllPortsSameDT=off  OutDataTypeStr=boolean
  Bitwise AND{,1..4} (5 alike) : simulink/Logic and Bit Operations/Bitwise Operator  logicop=AND  UseBitMask=on  BitMask=bin2dec('11111111')  BitMaskRealWorld=Stored Integer
  Bitwise AND10 : simulink/Logic and Bit Operations/Bitwise Operator  logicop=AND  UseBitMask=on  BitMask=bin2dec('00100000')  BitMaskRealWorld=Stored Integer
  Bitwise AND5 : simulink/Logic and Bit Operations/Bitwise Operator  logicop=AND  UseBitMask=on  BitMask=bin2dec('00000001')  BitMaskRealWorld=Stored Integer
  Bitwise AND6 : simulink/Logic and Bit Operations/Bitwise Operator  logicop=AND  UseBitMask=on  BitMask=bin2dec('00000010')  BitMaskRealWorld=Stored Integer
  Bitwise AND7 : simulink/Logic and Bit Operations/Bitwise Operator  logicop=AND  UseBitMask=on  BitMask=bin2dec('00000100')  BitMaskRealWorld=Stored Integer
  Bitwise AND8 : simulink/Logic and Bit Operations/Bitwise Operator  logicop=AND  UseBitMask=on  BitMask=bin2dec('00001000')  BitMaskRealWorld=Stored Integer
  Bitwise AND9 : simulink/Logic and Bit Operations/Bitwise Operator  logicop=AND  UseBitMask=on  BitMask=bin2dec('00010000')  BitMaskRealWorld=Stored Integer
  Bitwise OR2 : simulink/Logic and Bit Operations/Bitwise Operator  logicop=OR  UseBitMask=off  NumInputPorts=6  BitMask=bin2dec('00000000000000000000')  BitMaskRealWorld=Stored Integer
  Compare To Constant5 : simulink/Logic and Bit Operations/Compare To Constant  relop===  const=0  OutDataTypeStr=boolean
  Constant : Constant  OutDataTypeStr=uint8
  Constant1 : Constant  Value=2  OutDataTypeStr=uint8
  Constant2 : Constant  Value=3  OutDataTypeStr=uint8
  Constant3 : Constant  Value=4  OutDataTypeStr=uint8
  Constant4 : Constant  Value=5  OutDataTypeStr=uint8
  Constant5 : Constant  Value=7  OutDataTypeStr=uint8
  Data Type Conversion{,1..5} (6 alike) : DataTypeConversion  OutDataTypeStr=uint8
  Data Type Conversion{6..11} (6 alike) : DataTypeConversion  OutDataTypeStr=boolean
  Detect Change1 : simulink/Logic and Bit Operations/Detect Change  vinit=0  OutDataTypeStr=boolean
  Detect Increase : simulink/Logic and Bit Operations/Detect Increase  vinit=0.0  OutDataTypeStr=boolean
  Multiport Switch : MultiPortSwitch  Inputs=7  DataPortForDefault=Additional data port  DiagnosticForDefault=None
  NOT : Logic  Operator=NOT  IconShape=distinctive  AllPortsSameDT=off  OutDataTypeStr=boolean
  NOT1 : Logic  Operator=NOT  IconShape=distinctive  AllPortsSameDT=off  OutDataTypeStr=boolean
  Relational Operator{,1..5} (6 alike) : RelationalOperator  Operator===  OutDataTypeStr=boolean  RndMeth=Simplest
  Shift Arithmetic1 : ArithShift  BitShiftNumber=4  BitShiftDirection=Left
  Shift Arithmetic10 : ArithShift  BitShiftNumber=5  BitShiftDirection=Right
  Shift Arithmetic2 : ArithShift  BitShiftNumber=5  BitShiftDirection=Left
  Shift Arithmetic3 : ArithShift  BitShiftNumber=1  BitShiftDirection=Right
  Shift Arithmetic4 : ArithShift  BitShiftNumber=2  BitShiftDirection=Right
  Shift Arithmetic5 : ArithShift  BitShiftNumber=3  BitShiftDirection=Right
  Shift Arithmetic6 : ArithShift  BitShiftNumber=1  BitShiftDirection=Left
  Shift Arithmetic7 : ArithShift  BitShiftNumber=2  BitShiftDirection=Left
  Shift Arithmetic8 : ArithShift  BitShiftNumber=3  BitShiftDirection=Left
  Shift Arithmetic9 : ArithShift  BitShiftNumber=4  BitShiftDirection=Right
  Switch{,1..3,5,7,12..13} (8 alike) : Switch  Criteria=u2 ~= 0
  Switch{4,6,8..11} (6 alike) : Switch  Criteria=u2 > Threshold
  Unit Delay{1..4,6..14} (13 alike) : UnitDelay  SampleTime=-1  HasFrameUpgradeWarning=on
  Setting : Outport
  Set : Outport  Port=2
  wires:
  [Loadbar] -> AND/1
  Detect Increase/1 -> AND/2
  AND/1 -> Switch/2
  Unit Delay14/1 -> Switch12/3
  Unit Delay4/1 -> Switch12/2
  Unit Delay13/1 -> Switch13/3
  Unit Delay3/1 -> Switch13/2
  Unit Delay12/1 -> Switch7/3
  Unit Delay2/1 -> Switch7/2
  Unit Delay11/1 -> Switch5/3
  Unit Delay10/1 -> Switch5/2
  Unit Delay9/1 -> Switch3/2
  Unit Delay8/1 -> Switch2/2
  Unit Delay1/1 -> Switch3/3
  Unit Delay6/1 -> Switch2/3
  Relational Operator1/1 -> Unit Delay9/1
  Relational Operator/1 -> Unit Delay8/1
  [EEP_Set6] -> Switch11/3
  [EEP_Set5] -> Switch10/3
  [EEP_Set4] -> Switch9/3
  [EEP_Set3] -> Switch6/3
  [EEP_Set2] -> Switch4/3
  [EEP_Set1] -> Switch8/3
  Data Type Conversion11/1 -> [EEP_Set6]
  Data Type Conversion10/1 -> [EEP_Set5]
  Data Type Conversion9/1 -> [EEP_Set4]
  Data Type Conversion8/1 -> [EEP_Set3]
  Data Type Conversion7/1 -> [EEP_Set2]
  Data Type Conversion6/1 -> [EEP_Set1]
  [EEP_Set] -> Bitwise AND10/1
  [EEP_Set] -> Bitwise AND9/1
  [EEP_Set] -> Bitwise AND8/1
  [EEP_Set] -> Bitwise AND7/1
  [EEP_Set] -> Bitwise AND6/1
  [EEP_Set] -> Bitwise AND5/1
  EEP_Set/1 -> [EEP_Set]
  Shift Arithmetic5/1 -> Data Type Conversion9/1
  Shift Arithmetic9/1 -> Data Type Conversion10/1
  Bitwise AND7/1 -> Shift Arithmetic4/1
  Shift Arithmetic3/1 -> Data Type Conversion7/1
  Bitwise AND5/1 -> Data Type Conversion6/1
  Shift Arithmetic10/1 -> Data Type Conversion11/1
  Shift Arithmetic4/1 -> Data Type Conversion8/1
  Bitwise AND10/1 -> Shift Arithmetic10/1
  Bitwise AND9/1 -> Shift Arithmetic9/1
  Bitwise AND6/1 -> Shift Arithmetic3/1
  Bitwise AND8/1 -> Shift Arithmetic5/1
  Bitwise OR2/1 -> Set/1
  [Set3] -> Data Type Conversion2/1
  Bitwise AND4/1 -> Bitwise OR2/6
  Data Type Conversion1/1 -> Shift Arithmetic6/1
  Bitwise AND/1 -> Bitwise OR2/4
  [Set5] -> Data Type Conversion4/1
  [Set1] -> Data Type Conversion/1
  Data Type Conversion3/1 -> Shift Arithmetic8/1
  [Set2] -> Data Type Conversion1/1
  Data Type Conversion/1 -> Bitwise OR2/1
  [Set7] -> Data Type Conversion5/1
  Shift Arithmetic1/1 -> Bitwise AND3/1
  Shift Arithmetic7/1 -> Bitwise AND1/1
  Data Type Conversion4/1 -> Shift Arithmetic1/1
  Shift Arithmetic6/1 -> Bitwise AND2/1
  Bitwise AND2/1 -> Bitwise OR2/2
  Bitwise AND1/1 -> Bitwise OR2/3
  Bitwise AND3/1 -> Bitwise OR2/5
  Shift Arithmetic2/1 -> Bitwise AND4/1
  Shift Arithmetic8/1 -> Bitwise AND/1
  [Set4] -> Data Type Conversion3/1
  Data Type Conversion5/1 -> Shift Arithmetic2/1
  Data Type Conversion2/1 -> Shift Arithmetic7/1
  Relational Operator5/1 -> Unit Delay4/1
  Relational Operator4/1 -> Unit Delay3/1
  Relational Operator3/1 -> Unit Delay2/1
  Relational Operator2/1 -> Unit Delay10/1
  Unit Delay7/1 -> Switch1/1, [Set], NOT/1, Setting/1
  Switch11/1 -> Unit Delay14/1, [Set7]
  Switch12/1 -> Switch11/1
  Switch10/1 -> Unit Delay13/1, [Set5]
  Switch9/1 -> Unit Delay12/1, [Set4]
  Switch7/1 -> Switch9/1
  Switch5/1 -> Switch6/1
  Switch6/1 -> Unit Delay11/1, [Set3]
  Switch4/1 -> Unit Delay1/1, [Set2]
  Switch3/1 -> Switch4/1
  Switch2/1 -> Switch8/1
  Switch8/1 -> Unit Delay6/1, [Set1]
  Switch/1 -> Unit Delay7/1
  AND11/1 -> NOT1/1
  Compare To Constant5/1 -> AND11/1
  Constant4/1 -> Relational Operator4/2
  [Loadbar] -> Switch8/2
  [Set] -> Switch5/1
  [Loadbar] -> Switch6/2
  [Set] -> Switch7/1
  Constant1/1 -> Relational Operator1/2
  [UserNow] -> Relational Operator4/1
  [Set] -> Switch2/1
  Constant3/1 -> Relational Operator3/2
  [UserNow] -> Relational Operator3/1
  [UserNow] -> Relational Operator2/1
  [Loadbar] -> Switch9/2
  Constant/1 -> Relational Operator/2
  [Set] -> Switch3/1
  [Loadbar] -> Switch11/2
  Constant2/1 -> Relational Operator2/2
  [Loadbar] -> Switch10/2
  [UserNow] -> Relational Operator1/1
  [UserNow] -> Relational Operator/1
  Constant5/1 -> Relational Operator5/2
  [UserNow] -> Relational Operator5/1
  [Set] -> Switch12/1
  [Loadbar] -> Switch4/2
  [Set] -> Switch13/1
  iviCMD/1 -> Detect Increase/1
  NOT/1 -> Switch/1
  UserNow/1 -> Detect Change1/1, [UserNow], Multiport Switch/1
  Switch1/1 -> Switch/3
  Loadbar/1 -> Compare To Constant5/1, [Loadbar]
  Multiport Switch/1 -> Switch1/3
  Detect Change1/1 -> AND11/2
  Switch13/1 -> Switch10/1
  NOT1/1 -> Switch1/2
  [Set1] -> Multiport Switch/2
  [Set2] -> Multiport Switch/3
  [Set3] -> Multiport Switch/4
  [Set4] -> Multiport Switch/5
  [Set5] -> Multiport Switch/6
  [Set7] -> Multiport Switch/8
  Default/1 -> Multiport Switch/9, Multiport Switch/7
